simulink model "model"  (R2014b)
settings: Solver=ode45  SolverMode=SingleTasking  StartTime=0.0  StopTime=10  RelTol=1e-3
values from neighbouring files (symbols this model uses):
  A = [-0.32  -0.64; 1  0]    [ddddd.mat]
  B = [0.5 0;0 0.5;1 0;0 1]    [Final_exam_1.m]    (also in ddddd.mat = [1 0]; part1_Kalman.m)
  C = [0 1]    [ddddd.mat]
  Ec = 2236.06806909    [ddddd.mat]    (also in part2_Kalman.m = -inv(Co*inv(Ao-Bo*Kc)*Bo); part3_Kalman.m = -inv(Co*inv(Ao-Bo*Kc)*Bo); solver.m = -inv(Co*inv(Ao-Bo*Kc)*Bo))
  Kc = [66.5452266741 2235.42806909]    [ddddd.mat]
  L = [50.749673304 71.42478104]    [ddddd.mat]    (also in part2_Kalman.m = Ko; part3_Kalman.m = Ko)
  laserAngle = [3.0505359435 3.05311711406 3.05396640859 3.05214394079 3.05005181397 3.04988530837 3.05048038439 3.0515938321 3.05152009387 3.05057608588 3.05074155154 3.04987957951 ... (851 elements, 1x851)]    [ddddd.mat]    (also in laserAngle.mat = [3.0505359435 3.05310955561 3.05396213531 3.05216158176 3.05)
  xo_ini = [0.5 0.5]    [ddddd.mat]    (also in part2_Kalman.m = [ 0.5  ; 0.5 ]; part3_Kalman.m = [ 1  ; 1 ]; solver.m = [ 0.5  ; 0.5 ])
settings Model: CovSFcnEnable=on  Creator=user  LastModifiedBy=123
settings OptimizationCC: BlockReduction=off  BooleanDataType=off  UseDivisionForNetSlopeComputation=off  SimCompilerOptimization=off
settings DebuggingCC: SaveWithParameterizedLinksMsg=none  UnderspecifiedInitializationDetection=Classic  MergeDetectMultiDrivingBlocksExec=none  SignalResolutionControl=TryResolveAllWithWarning  SolverPrmCheckMsg=none  FrameProcessingCompatibilityMsg=error
settings HardwareCC: TargetUnknown=on
settings RTWCC: RTWCompilerOptimization=off

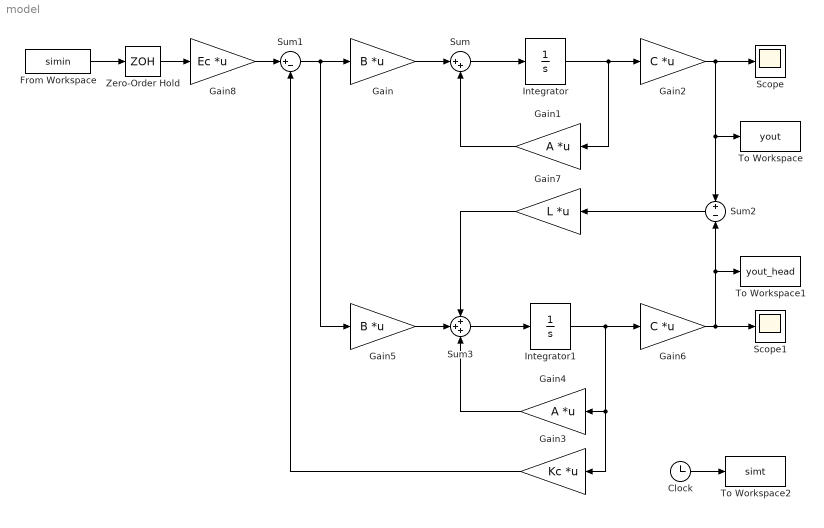
== system model ==
  Clock : Clock
  From Workspace : FromWorkspace  VariableName=simin  SampleTime=0
  Gain : Gain  Gain=B  Multiplication=Matrix(K*u)
  Gain1 : Gain  Gain=A  Multiplication=Matrix(K*u)
  Gain2 : Gain  Gain=C  Multiplication=Matrix(K*u)
  Gain3 : Gain  Gain=Kc  Multiplication=Matrix(K*u)
  Gain4 : Gain  Gain=A  Multiplication=Matrix(K*u)
  Gain5 : Gain  Gain=B  Multiplication=Matrix(K*u)
  Gain6 : Gain  Gain=C  Multiplication=Matrix(K*u)
  Gain7 : Gain  Gain=L  Multiplication=Matrix(K*u)
  Gain8 : Gain  Gain=Ec  Multiplication=Matrix(K*u)
  Integrator : Integrator  InitialCondition=laserAngle(1)
  Integrator1 : Integrator  InitialCondition=xo_ini
  Scope : Scope
  Scope1 : Scope
  Sum : Sum  Inputs=|++
  Sum1 : Sum  Inputs=|+-
  Sum2 : Sum  Inputs=+|-
  Sum3 : Sum  Inputs=+++
  To Workspace : ToWorkspace  VariableName=yout  SampleTime=-1
  To Workspace1 : ToWorkspace  VariableName=yout_head  SampleTime=-1
  To Workspace2 : ToWorkspace  VariableName=simt  SampleTime=-1
  Zero-Order Hold : ZeroOrderHold
  wires:
  Gain/1 -> Sum/1
  Gain1/1 -> Sum/2
  Sum/1 -> Integrator/1
  Integrator/1 -> Gain2/1, Gain1/1
  Sum1/1 -> Gain5/1, Gain/1
  Gain2/1 -> Sum2/1, To Workspace/1, Scope/1
  Clock/1 -> To Workspace2/1
  Integrator1/1 -> Gain6/1, Gain3/1, Gain4/1
  Gain6/1 -> Scope1/1, Sum2/2, To Workspace1/1
  Gain7/1 -> Sum3/1
  Gain5/1 -> Sum3/2
  Gain4/1 -> Sum3/3
  Sum3/1 -> Integrator1/1
  Sum2/1 -> Gain7/1
  From Workspace/1 -> Zero-Order Hold/1
  Gain8/1 -> Sum1/1
  Gain3/1 -> Sum1/2
  Zero-Order Hold/1 -> Gain8/1
